simulink model "simulink_rover_control"  (R2021b)
settings: Solver=FixedStepAuto  StartTime=0.0  StopTime=inf  RelTol=1e-3  EnableMultiTasking=on
model workspace (MAT data in the model file):
  ON = 1
libraries: arduinomotorcarrierlib x6, arduinolib x1
settings Model: ExtModeTrigDuration=2  Creator=ssekar  LastModifiedBy=sduraira
settings OptimizationCC: EnhancedBackFolding=on  PassReuseOutputArgsAs=Individual arguments  ZeroExternalMemoryAtStartup=off  ZeroInternalMemoryAtStartup=off  MaxStackSize=64  OptimizeBlockOrder=speed  DifferentSizesBufferReuse=on  OptimizationCustomize=off  EfficientTunableParamExpr=on
settings DebuggingCC: ParameterPrecisionLossMsg=none  ParameterTunabilityLossMsg=error
settings HardwareCC: ProdBitPerPointer=32  ProdBitPerSizeT=32  ProdBitPerPtrDiffT=32  ProdLargestAtomicInteger=Long  ProdLargestAtomicFloat=Double  ProdWordSize=32  ProdHWDeviceType=ARM Compatible->ARM Cortex
settings SFSimCC: MATLABDynamicMemAlloc=off
settings RTWCC: Description=Embedded Coder  SystemTargetFile=ert.tlc  HardwareBoard=Arduino Nano 33 IoT  TemplateMakefile=ert_default_tmf  Toolchain=Arduino ARM  BuildConfiguration=Faster Runs
settings CodeAppCC: ForceParamTrailComments=on  IgnoreCustomStorageClasses=off  OperatorAnnotations=on  SimulinkDataObjDesc=on  SFDataObjDesc=on  InsertBlockDesc=on
settings ERTTargetCC: SupportContinuousTime=on  SupportVariableSizeSignals=on  ExtModeTransport=3  ExtModeStaticAlloc=on  ExtModeStaticAllocSize=8192  ExtModeMexFile=ext_xcp  ExtModeIntrfLevel=Level2 - Open

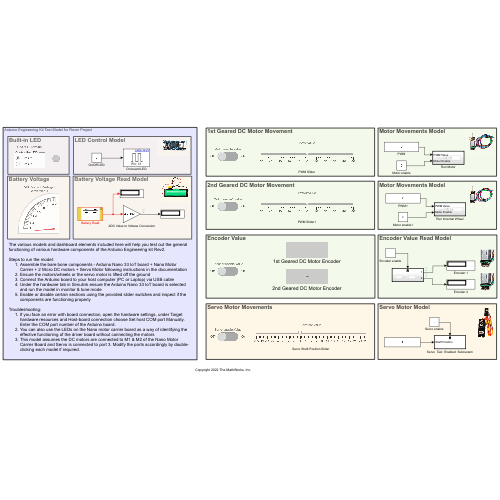
[thumbnail: Simulink's stored preview of the top-level diagram]
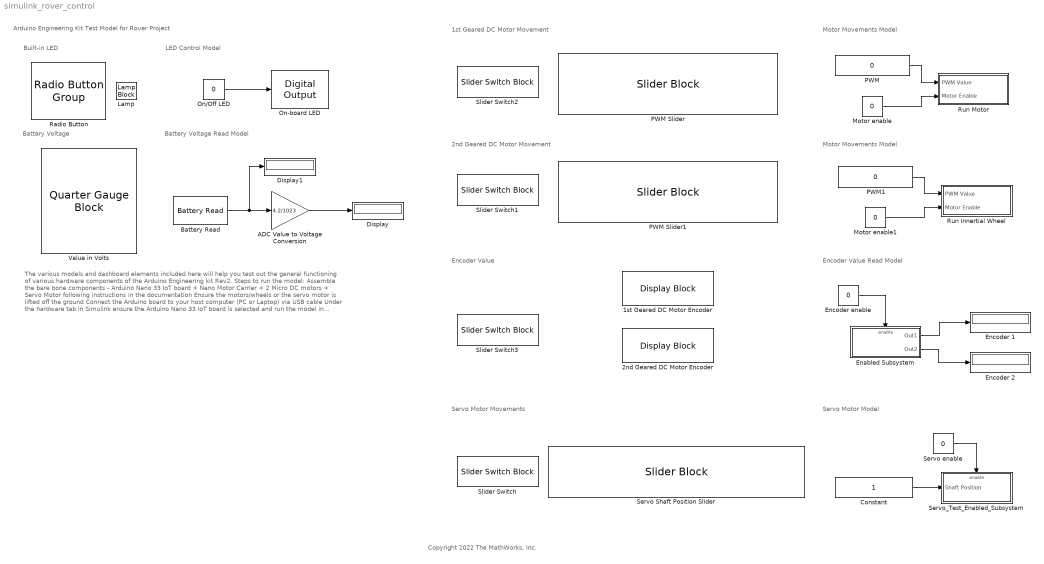
== system simulink_rover_control ==
  note: The various models and dashboard elements included here will help you test out the general functioning of various hardware components of the Arduino Engineering kit Rev2.
      |
      | Steps to run the model:
      | Assemble the bare bone components - Arduino Nano 33 IoT board + Nano Motor Carrier + 2 Micro DC motors + Servo Motor following instructions in the documentation
      | Ensure the motors/wheels or the servo motor is lifted off the ground
      | Connect the Arduino board to your host computer (PC or Laptop) via USB cable
      | Under the hardware tab in Simulink ensure the Arduino Nano 33 IoT board is selected and run the model in monitor & tune mode
      | Enable or disable certain sections using the provided slider switches and inspect if the components are functioning properly
      |
      | Troubleshooting:
      | If you face an error with board connection, open the hardware settings, under Target hardware resources and Host-board connection choose Set host COM port Manually. Enter the COM port number of the Arduino board.
      | You can also use the LEDs on the Nano motor carrier board as a way of identifying the effective functioning of the driver board without connecting the motors
      | This model assumes the DC motors are connected to M1 & M2 of the Nano Motor Carrier Board and Servo is connected to port 3. Modify the ports accordingly by double-clicking each model if required.
  note: Arduino Engineering Kit Test Model for Rover Project
  note: Motor Movements Model
  note: Encoder Value Read Model
  note: Battery Voltage Read Model
  note: Servo Motor Model
  note: LED Control Model
  note: Encoder Value
  note: 2nd Geared DC Motor Movement
  note: Servo Motor Movements
  note: Battery Voltage
  note: Built-in LED
  note: Copyright 2022 The MathWorks, Inc.
  note: Motor Movements Model
  note: 1st Geared DC Motor Movement
  1st Geared DC Motor Encoder : DisplayBlock  LabelPosition=Hide  Format=short  Transparency=1
  2nd Geared DC Motor Encoder : DisplayBlock  LabelPosition=Hide  Format=short  Transparency=1
  ADC Value to Voltage Conversion : Gain  Gain=4.2/1023
  Battery Read : arduinomotorcarrierlib/Battery Read  SlaveAddress=uint8( hex2dec( '66' ) )  blockPlatform=ARDUINO  SampleTime=-1
      settings: SourceProductBaseCode=ARDUINO
  Constant : Constant
  Display : Display
  Display1 : Display
  Enabled Subsystem : Subsystem  TreatAsAtomicUnit=on
  Encoder 1 : Display
  Encoder 2 : Display
  Encoder enable : Constant  Value=0
  Lamp : LampBlock  LabelPosition=Hide
  Motor enable : Constant  Value=0
  Motor enable1 : Constant  Value=0
  On-board LED : arduinolib/Digital Output  pinNumber=13  Direction=output  blockPlatform=arduino
  On/Off LED : Constant  Value=0
  PWM : Constant  Value=0
  PWM Slider : SliderBlock  ScaleMin=-50  ScaleMax=50  TickInterval=10
  PWM Slider1 : SliderBlock  ScaleMin=-50  ScaleMax=50  TickInterval=10
  PWM1 : Constant  Value=0
  Radio Button : RadioButtonGroup  SelectedLabel=Turn Off  ButtonGroupName=Control the LED
      settings: Values={{'Turn Off', 'Turn On'}, [0 1]}
  Run Innertial Wheel : Subsystem  TreatAsAtomicUnit=on
  Run Motor : Subsystem  TreatAsAtomicUnit=on
  Servo Shaft Position Slider : SliderBlock  ScaleMin=-15  ScaleMax=25  TickInterval=2
  Servo enable : Constant  Value=0
  Servo_Test_Enabled_Subsystem : Subsystem  TreatAsAtomicUnit=on
  Slider Switch{,1..3} (4 alike) : SliderSwitchBlock
      settings: Values={{'Off', 'On'}, [0 1]}
  Value in Volts : QuarterGaugeBlock  ScaleMin=3  ScaleMax=4.2  TickInterval=0.2
  wires:
  ADC Value to Voltage Conversion/1 -> Display/1
  Battery Read/1 -> Display1/1, ADC Value to Voltage Conversion/1
  Encoder enable/1 -> Enabled Subsystem/Enable
  Enabled Subsystem/1(Out1) -> Encoder 1/1
  Enabled Subsystem/2(Out2) -> Encoder 2/1
  Servo enable/1 -> Servo_Test_Enabled_Subsystem/Enable
  On/Off LED/1 -> On-board LED/1
  Constant/1 -> Servo_Test_Enabled_Subsystem/1(Shaft Position)
  PWM/1 -> Run Motor/1(PWM Value)
  Motor enable/1 -> Run Motor/2(Motor Enable)
  Motor enable1/1 -> Run Innertial Wheel/2(Motor Enable)
  PWM1/1 -> Run Innertial Wheel/1(PWM Value)

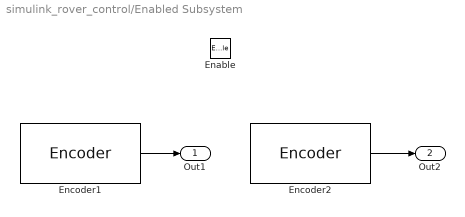
== system simulink_rover_control/Enabled Subsystem ==
  Enable : EnablePort
  Encoder1 : arduinomotorcarrierlib/Encoder  SlaveAddress=uint8( hex2dec( '66' ) )  blockPlatform=ARDUINO  Encoder=1  ShowSpeed=off  ResetOption=on  SampleTime=0.1
      settings: SourceProductBaseCode=ARDUINO
  Encoder2 : arduinomotorcarrierlib/Encoder  SlaveAddress=uint8( hex2dec( '66' ) )  blockPlatform=ARDUINO  Encoder=2  ShowSpeed=off  ResetOption=on  SampleTime=0.1
      settings: SourceProductBaseCode=ARDUINO
  Out1 : Outport
  Out2 : Outport  Port=2
  wires:
  Encoder1/1 -> Out1/1
  Encoder2/1 -> Out2/1

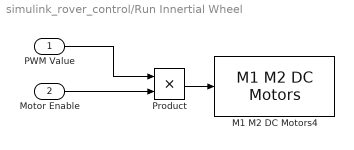
== system simulink_rover_control/Run Innertial Wheel ==
  PWM Value : Inport
  Motor Enable : Inport  Port=2
  M1 M2 DC Motors4 : arduinomotorcarrierlib/M1 M2 DC Motors  SlaveAddress=uint8( hex2dec( '66' ) )  blockPlatform=ARDUINO  MotorNumber=M2  MotorCarrierPWMFreq=100
      settings: SourceProductBaseCode=ARDUINO
  Product : Product
  wires:
  Product/1 -> M1 M2 DC Motors4/1
  PWM Value/1 -> Product/1
  Motor Enable/1 -> Product/2

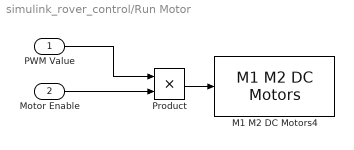
== system simulink_rover_control/Run Motor ==
  PWM Value : Inport
  Motor Enable : Inport  Port=2
  M1 M2 DC Motors4 : arduinomotorcarrierlib/M1 M2 DC Motors  SlaveAddress=uint8( hex2dec( '66' ) )  blockPlatform=ARDUINO  MotorNumber=M1  MotorCarrierPWMFreq=100
      settings: SourceProductBaseCode=ARDUINO
  Product : Product
  wires:
  Product/1 -> M1 M2 DC Motors4/1
  PWM Value/1 -> Product/1
  Motor Enable/1 -> Product/2

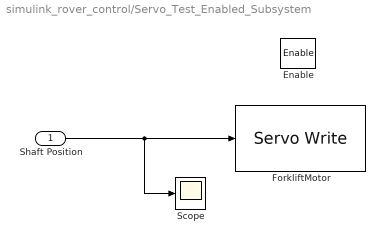
== system simulink_rover_control/Servo_Test_Enabled_Subsystem ==
  Shaft Position : Inport
  Enable : EnablePort
  ForkliftMotor : arduinomotorcarrierlib/Servo Write  SlaveAddress=uint8( hex2dec( '66' ) )  blockPlatform=ARDUINO  MotorNumber=3  MotorCarrierPWMFreq=100
      settings: SourceProductName=Simulink Support for Arduino MKR Motor Carrier
  Scope : Scope
  wires:
  Shaft Position/1 -> Scope/1, ForkliftMotor/1
